simulink model "pmsg_wind_turbine"  (R2022a)
settings: Solver=ode23tb  StartTime=0.0  StopTime=30  FixedStep=1e-4  MaxStep=1e-4  RelTol=1e-3
undefined symbols (not defined in the file): Ci, kde, ke, Lb, sigbuilder_block, time, vwind
libraries: spsCurrentMeasurementLib x3, spsVoltageMeasurementLib x3, fuzblock x2, spsPWMGeneratorDCDCLib x2, eePowerMeasurement x2, spsSeriesRLCBranchLib x2, spsDCVoltageSourceLib x1, spsDiodeLib x1, spsMosfetLib x1, spsPermanentMagnetSynchronousMachineLib x1, spsThreePhaseVIMeasurementLib x1, spsUniversalBridgeLib x1
settings Model: Creator=Taysa Banik  LastModifiedBy=LICON
settings SolverCC: ZeroCrossAlgorithm=Adaptive
settings DebuggingCC: MaxConsecutiveZCsMsg=warning  MaskedZcDiagnostic=none  IgnoredZcDiagnostic=none  MultiTaskCondExecSysMsg=warning  MultiTaskRateTransMsg=warning  ModelReferenceExtraNoncontSigs=warning

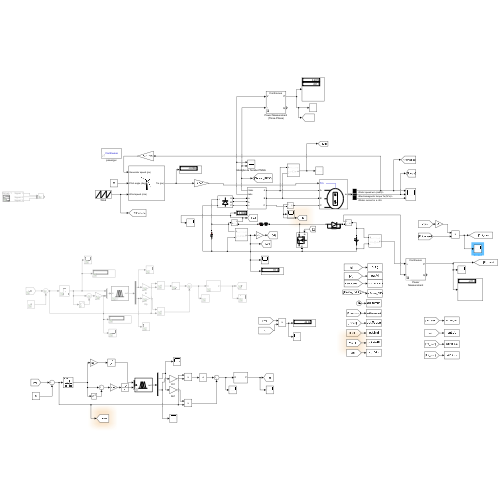
[thumbnail: Simulink's stored preview of the top-level diagram]
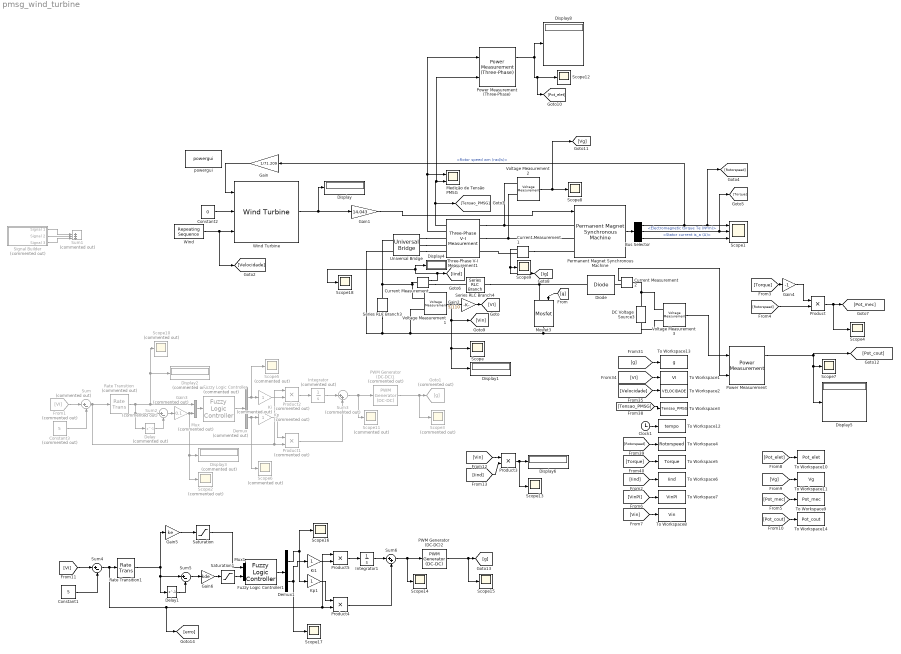
== system pmsg_wind_turbine ==
  Bus Selector : BusSelector  OutputSignals=Rotor speed wm (rad/s),Electromagnetic torque Te (N*m),Stator current is_a (A)
  Clock1 : Clock
  Constant1 : Constant  Value=5
  Constant2 : Constant  Value=0
  Constant3 : Constant  Commented=on  Value=5
  Current Measurement : spsCurrentMeasurementLib/Current Measurement  PhasorSimulation=off  OutputType=Complex  PSBequivalent=0
  Current Measurement1 : spsCurrentMeasurementLib/Current Measurement  PhasorSimulation=off  OutputType=Complex  PSBequivalent=0
  Current Measurement2 : spsCurrentMeasurementLib/Current Measurement  PhasorSimulation=off  OutputType=Complex  PSBequivalent=0
  DC Voltage Source3 : spsDCVoltageSourceLib/DC Voltage Source  Amplitude=400  Measurements=None
  Delay : Delay  Commented=on  DelayLength=1
  Delay1 : Delay  DelayLength=1
  Demux : Demux  Commented=on  Outputs=2
  Demux1 : Demux  Outputs=2
  Diode : spsDiodeLib/Diode  Ron=0.001  Lon=0  Vf=0.1  IC=0  UseSnubber=0  Rs=50000  Cs=inf  Measurements=off
  Display{,1,4..6,8} (6 alike) : Display
  Display2 : Display  Commented=on
  Display3 : Display  Commented=on
  From1 : From  Commented=on  GotoTag=VI
  Fuzzy Logic Controller : fuzblock/Fuzzy Logic  Controller  Commented=on  FIS=controladormppt  OutputSampleNumber=101  DataType=double  FuzzifiedInputs=off  RuleFiringStrengths=off  RuleOutputs=off  AggregatedOutputs=off  SimulateUsing=Interpreted execution  OutOfRangeInputValueMessage=warning  NoRuleFiredMessage=warning  EmptyOutputFuzzySetMessage=warning
  Fuzzy Logic Controller1 : fuzblock/Fuzzy Logic  Controller  FIS=controladormppt  OutputSampleNumber=101  DataType=double  FuzzifiedInputs=off  RuleFiringStrengths=off  RuleOutputs=off  AggregatedOutputs=off  SimulateUsing=Interpreted execution  OutOfRangeInputValueMessage=warning  NoRuleFiredMessage=warning  EmptyOutputFuzzySetMessage=warning
  Gain : Gain  Gain=1/71.209
  Gain1 : Gain  Gain=14.043
  Gain2 : Gain  Gain=5/110
  Gain3 : Gain  Commented=on  Gain=0.1
  Gain4 : Gain  Gain=-1
  Gain5 : Gain  Gain=ke
  Gain6 : Gain  Gain=kde
  Goto1 : Goto  Commented=on  GotoTag=g
  Integrator : Integrator  Commented=on
  Integrator1 : Integrator
  Ki : Gain  Commented=on
  Ki1 : Gain
  Kp : Gain  Commented=on
  Kp1 : Gain
  Medição de Tensão PMSG : Scope  NumInputPorts=2
  Mosfet3 : spsMosfetLib/Mosfet  Ron=0.001  Lon=0  Rd=0.01  Vfd=0  IC=0  Rs=1e5  Cs=inf  Measurements=off
  Mux : Mux  Commented=on  Inputs=2
  Mux1 : Mux  Inputs=2
  PWM Generator (DC-DC)1 : spsPWMGeneratorDCDCLib/PWM Generator (DC-DC)  Commented=on  Fsw=30000  Ts=1e-6
  PWM Generator (DC-DC)2 : spsPWMGeneratorDCDCLib/PWM Generator (DC-DC)  Fsw=30000  Ts=1e-6
  Permanent Magnet Synchronous Machine : spsPermanentMagnetSynchronousMachineLib/Permanent Magnet Synchronous Machine  NbPhases=3  FluxDistribution=Sinusoidal  RotorType=Round  MechanicalLoad=Torque Tm  PresetModel=No  ShowDetailedParameters=on  MeasurementBus=off  Resistance=0.732  Inductance=8.5e-3  dqInductances=[8.5e-3,8.5e-3]  La=3.8e-3  MachineConstant=Voltage Constant (V_peak L-L / krpm)  Flux=0.13618  VoltageCst=172.9  TorqueCst=1.4299  Flat=120  Mechanical=[1e-3 1.79E-4 7 0]  PolePairs=4  InitialConditions=[71.21,0, 0,0]  InitialConditions5ph=[0 0 0 0 0 0]  RefAngle=Aligned with phase A axis (original Park)  IterativeDiscreteModel=Trapezoidal non iterative  TsBlock=-1  TsPowergui=0
  Power Measurement : eePowerMeasurement/Power Measurement  LabelModeActiveChoice=Continuous  F=79.33  K=[0]  Ts=0
      settings: SourceProductBaseCode=PS
  Power Measurement (Three-Phase) : eePowerMeasurement/Power Measurement (Three-Phase)  LabelModeActiveChoice=Continuous  F=79.33  K=[0 1]  Seq=Positive  Ts=0
      settings: SourceProductBaseCode=PS
  Product{,3..5} (4 alike) : Product
  Product1 : Product  Commented=on
  Product2 : Product  Commented=on
  Rate Transition : RateTransition  Commented=on  OutPortSampleTime=1e-4
  Rate Transition1 : RateTransition  OutPortSampleTime=1e-4
  Saturation : Saturate  UpperLimit=1  LowerLimit=-1
  Saturation1 : Saturate  UpperLimit=1  LowerLimit=-1
  Scope{,4,7..9,12..18} (12 alike) : Scope
  Scope1 : Scope  NumInputPorts=3
  Scope{2..3,5..6,10..11} (6 alike) : Scope  Commented=on
  Series RLC Branch3 : spsSeriesRLCBranchLib/Series RLC Branch  LConnTagsString=__new0  RConnTagsString=__new0  BranchType=C  Resistance=1  Inductance=1e-3  SetiL0=off  InitialCurrent=0  Capacitance=Ci  Setx0=on  InitialVoltage=100  Measurements=None
  Series RLC Branch4 : spsSeriesRLCBranchLib/Series RLC Branch  LConnTagsString=__new0  RConnTagsString=__new0  BranchType=RL  Resistance=1  Inductance=Lb  SetiL0=off  InitialCurrent=0  Capacitance=1e-3  Setx0=off  InitialVoltage=0  Measurements=None
  Signal Builder : Subsystem  Tag=STV Subsys  Commented=on  LoadFcn=sigbuilder_block('load');  StartFcn=sigbuilder_block('start');  StopFcn=sigbuilder_block('stop');  ClipboardFcn=sigbuilder_block('clipboard');  mask(Sigbuilder block){tuvar=[0:10]}
      mask help: Simulink:masks:SigbuilderBlock_MD
      mask init:
      | if ~strcmp(get_param(bdroot(gcbh),'SimulationStatus'),'stopped') tuvar = sigbuilder_block('maskInit'); end
      settings: CopyFcn=sigbuilder_block('copy');  DeleteFcn=sigbuilder_block('delete');  ModelCloseFcn=sigbuilder_block('modelClose');  PreSaveFcn=sigbuilder_block('preSave');  PauseFcn=sigbuilder_block('pause');  ContinueFcn=sigbuilder_block('continue');  NameChangeFcn=sigbuilder_block('namechange');  OpenFcn=sigbuilder_block('open',[61.5 90 1012.5 506.25 ]);  CloseFcn=sigbuilder_block('close');
      mask Display: plot(0, 0, 100, 100,[2, 2, 32, 32, 2], [68, 8, 8, 68, 68],[32, 2], [38, 38], [32, 19, 2],[53, 60, 44], [32, 17, 17, 2],[16, 16, 31, 31]);txt = getActiveGroup(gcbh);text(2, 100, txt,'verticalAlignment', 'top');
  Sum : Sum  Commented=on  Inputs=|+-
  Sum1 : Sum  Commented=on  Inputs=|+++
  Sum2 : Sum  Commented=on  Inputs=|+-
  Sum3 : Sum  Commented=on  Inputs=|++
  Sum4 : Sum  Inputs=|+-
  Sum5 : Sum  Inputs=|+-
  Sum6 : Sum  Inputs=|++
  Three-Phase V-I Measurement1 : spsThreePhaseVIMeasurementLib/Three-Phase V-I Measurement  VoltageMeasurement=phase-to-phase  SetLabelV=off  LabelV=Vabc  Vpu=off  VpuLL=off  CurrentMeasurement=yes  SetLabelI=off  LabelI=Iabc  Ipu=off  Pbase=100e6  Vbase=500e3  OutputType=Complex  PhasorSimulation=off  PSBequivalent=0
  To Workspace1 : ToWorkspace  VariableName=VI  SampleTime=1e-6
  To Workspace10 : ToWorkspace  VariableName=Pot_elet  SampleTime=1e-6
  To Workspace11 : ToWorkspace  VariableName=Vg  SampleTime=1e-6
  To Workspace12 : ToWorkspace  VariableName=tempo  SampleTime=1e-6
  To Workspace13 : ToWorkspace  VariableName=g  SampleTime=1e-6
  To Workspace14 : ToWorkspace  VariableName=Pot_cout  SampleTime=1e-6
  To Workspace2 : ToWorkspace  VariableName=VELOCIDADE  SampleTime=1e-6
  To Workspace3 : ToWorkspace  VariableName=Tensao_PMSG  SampleTime=1e-6
  To Workspace4 : ToWorkspace  VariableName=Rotorspeed  SampleTime=1e-6
  To Workspace5 : ToWorkspace  VariableName=Torque  SampleTime=1e-6
  To Workspace6 : ToWorkspace  VariableName=Iind  SampleTime=1e-6
  To Workspace7 : ToWorkspace  VariableName=VinPI  SampleTime=1e-6
  To Workspace8 : ToWorkspace  VariableName=Vin  SampleTime=1e-6
  To Workspace9 : ToWorkspace  VariableName=Pot_mec  SampleTime=1e-6
  Universal Bridge : spsUniversalBridgeLib/Universal Bridge  Arms=3  SnubberResistance=1e5  SnubberCapacitance=inf  Device=Diodes  Ron=1e-3  Lon=0  ForwardVoltages="[  0  0  ]"  ForwardVoltage=0.1  GTOparameters=[ 10e-6 , 20e-6 ]  IGBTparameters=[ 1e-6 , 2e-6 ]  Measurements=None  Measurements_2=None  converterType=Rectifier
  Voltage Measurement1 : spsVoltageMeasurementLib/Voltage Measurement  PhasorSimulation=off  OutputType=Complex  PSBequivalent=0
  Voltage Measurement2 : spsVoltageMeasurementLib/Voltage Measurement  PhasorSimulation=off  OutputType=Complex  PSBequivalent=0
  Voltage Measurement3 : spsVoltageMeasurementLib/Voltage Measurement  PhasorSimulation=off  OutputType=Complex  PSBequivalent=0
  Wind : simulink/Sources/Repeating Sequence  rep_seq_t=[time]  rep_seq_y=[vwind]
  Wind Turbine : spsWindTurbineLib/Wind Turbine  Pnom=1000  Pelec_base=1000  wind_base=12  P_wind_base=1  speed_nom=1  pitch_angle=0  c1_c6="[0.51763          116          0.4            5           21     0.006795]"  cp_nom=0.48  lambda_nom=8.1
      settings: SourceProductBaseCode=PS
  powergui : spspowerguiLib/powergui  Priority=1  SimulationMode=Continuous  SampleTime=50e-6  frequency=60  Iterations=50  frequencyindice=0  Pbase=100e6  ErrMax=1e-4  UnitsV=kV  UnitsW=MW  buscounter=0  FunctionMessages=off  echomessages=off  EnableUseOfTLC=off  CurrentSourceSwitches=off  DisableSnubberDevices=off  DisableRonSwitches=off  DisableVfSwitches=off  DisplayEquations=off  AutomaticDiscreteSolvers=off  SolverType=Tustin/Backward Euler (TBE)  Interpol=off  ExternalGateDelay=off  methode=off  Ts=100  x0status=blocks  SPID=on  SwTol=0  HookPort=off  NonlinearTolerance=1e-4  nMaxIteration=100  ContinueOnMaxIteration=off  RestoreLinks=warning  ResistiveCurrentMeasurement=off  Frange=[0:2:500]  Ylog=off  Xlog=on  ShowGrid=off  save=off  variable=ZData  structure=0  ZoomFFT=off  StartTime=0.0  cycles=1  DisplayStyle=1  fundamental=60  FreqAxis=off  MaxFrequency=1000  frequencyindicesteady=1  RmsSteady=1  display=off
  wires:
  Constant2/1 -> Wind Turbine/2
  Three-Phase V-I Measurement1/1 -> Power Measurement (Three-Phase)/2, Medição de Tensão PMSG/2, [Tensao_PMSG]
  Three-Phase V-I Measurement1/2 -> Power Measurement (Three-Phase)/1, Medição de Tensão PMSG/1
  Permanent Magnet Synchronous Machine/1 -> Bus Selector/1
  Bus Selector/1 -> Scope1/1, [Rotorspeed], Gain/1  "<Rotor speed wm (rad/s)>"
  Bus Selector/2 -> [Torque], Scope1/2  "<Electromagnetic torque Te (N*m)>"
  Bus Selector/3 -> Scope1/3  "<Stator current is_a (A)>"
  Gain/1 -> Wind Turbine/1
  Wind Turbine/1 -> Display/1, Gain1/1
  Gain1/1 -> Permanent Magnet Synchronous Machine/1
  Voltage Measurement1/1 -> Gain2/1, Scope/1, Display1/1, [Vin]
  [g] -> Mosfet3/1
  From1/1 -> Sum/1
  Constant3/1 -> Sum/2
  PWM Generator (DC-DC)1/1 -> Scope3/1, Goto1/1
  Gain2/1 -> [VI]
  Signal Builder/1(Signal 1) -> Sum1/1
  Signal Builder/2(Signal 2) -> Sum1/2
  Signal Builder/3(Signal 3) -> Sum1/3
  [VI] -> To Workspace1/1
  [g] -> To Workspace13/1
  [Torque] -> To Workspace5/1
  [Velocidade] -> To Workspace2/1
  Clock1/1 -> To Workspace12/1
  [Tensao_PMSG] -> To Workspace3/1
  [Rotorspeed] -> To Workspace4/1
  Current Measurement/1 -> Scope18/1, Display4/1, [Iind]
  [Iind] -> To Workspace6/1
  Product/1 -> Scope4/1, [Pot_mec]
  [Rotorspeed] -> Product/2
  [Torque] -> Gain4/1
  Gain4/1 -> Product/1
  Sum/1 -> Rate Transition/1, Product2/1, Product1/2
  Demux/2 -> Scope6/1, Kp/1
  Kp/1 -> Product1/1
  Demux/1 -> Scope5/1, Ki/1
  Ki/1 -> Product2/2
  Product2/1 -> Integrator/1
  Integrator/1 -> Sum3/1
  Product1/1 -> Sum3/2
  Sum3/1 -> Scope11/1, PWM Generator (DC-DC)1/1
  Mux/1 -> Fuzzy Logic Controller/1
  Fuzzy Logic Controller/1 -> Demux/1
  [VinPI] -> To Workspace7/1
  [Vin] -> To Workspace8/1
  [Pot_mec] -> To Workspace9/1
  [Pot_elet] -> To Workspace10/1
  Voltage Measurement2/1 -> [Vg], Scope8/1
  Current Measurement1/1 -> [Ig], Scope9/1
  [Vg] -> To Workspace11/1
  Power Measurement (Three-Phase)/1 -> [Pot_elet], Scope12/1, Display8/1
  Power Measurement/1 -> Display5/1, Scope7/1, [Pot_cout]
  Voltage Measurement3/1 -> Power Measurement/1
  Current Measurement2/1 -> Power Measurement/2
  [Pot_cout] -> To Workspace14/1
  Gain3/1 -> Scope2/1, Display3/1, Mux/2
  Rate Transition/1 -> Delay/1, Sum2/1, Scope10/1, Display2/1, Mux/1
  Sum2/1 -> Gain3/1
  Delay/1 -> Sum2/2
  [Iind] -> Product3/2
  Product3/1 -> Scope13/1, Display6/1
  [Vin] -> Product3/1
  Saturation1/1 -> Mux1/2
  Sum5/1 -> Gain6/1
  Delay1/1 -> Sum5/2
  Integrator1/1 -> Sum6/1
  Mux1/1 -> Fuzzy Logic Controller1/1
  Demux1/1 -> Kp1/1, Scope16/1
  Gain5/1 -> Saturation/1
  Ki1/1 -> Product5/2
  Sum6/1 -> Scope14/1, PWM Generator (DC-DC)2/1
  Rate Transition1/1 -> Gain5/1, Delay1/1, Sum5/1
  Constant1/1 -> Sum4/2
  [VI] -> Sum4/1
  Demux1/2 -> Ki1/1, Scope17/1
  PWM Generator (DC-DC)2/1 -> Scope15/1, [g]
  Product5/1 -> Integrator1/1
  Sum4/1 -> Rate Transition1/1, [erro], Product5/1, Product4/2
  Saturation/1 -> Mux1/1
  Gain6/1 -> Saturation1/1
  Kp1/1 -> Product4/1
  Product4/1 -> Sum6/2
  Fuzzy Logic Controller1/1 -> Demux1/1
  Wind/1 -> [Velocidade], Wind Turbine/3
  connections:
  Three-Phase V-I Measurement1/LConn1 -- Voltage Measurement2/LConn1 -- Permanent Magnet Synchronous Machine/LConn1
  Three-Phase V-I Measurement1/LConn2 -- Voltage Measurement2/LConn2 -- Permanent Magnet Synchronous Machine/LConn2
  Universal Bridge/LConn1 -- Three-Phase V-I Measurement1/RConn1
  Universal Bridge/LConn2 -- Three-Phase V-I Measurement1/RConn2
  Universal Bridge/LConn3 -- Three-Phase V-I Measurement1/RConn3
  Mosfet3/LConn1 -- Diode/LConn1 -- Series RLC Branch4/RConn1
  Voltage Measurement1/LConn1 -- Current Measurement/LConn1 -- Universal Bridge/RConn1 -- Series RLC Branch3/LConn1
  Series RLC Branch3/RConn1 -- Universal Bridge/RConn2 -- Voltage Measurement1/LConn2 -- Voltage Measurement3/LConn2 -- DC Voltage Source3/LConn1 -- Mosfet3/RConn1
  DC Voltage Source3/RConn1 -- Current Measurement2/LConn1 -- Voltage Measurement3/LConn1
  Current Measurement1/LConn1 -- Permanent Magnet Synchronous Machine/LConn3
  Current Measurement1/RConn1 -- Three-Phase V-I Measurement1/LConn3
  Current Measurement2/RConn1 -- Diode/RConn1
  Current Measurement/RConn1 -- Series RLC Branch4/LConn1

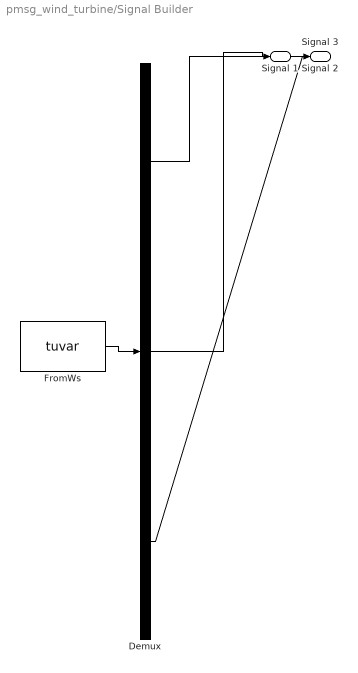
== system pmsg_wind_turbine/Signal Builder ==
  Demux : Demux  Tag=STV Demux  Outputs=3
      settings: DisplayOption=none
  FromWs : FromWorkspace  Tag=STV FromWs  VariableName=tuvar
      SigBuilderData=|
      | common.afterFinalStr = 'Extrapolate'
      | common.sampleTime = 0
      | dataSet.timeRange = [0 10]
      | dataSet.name = 'Group 1'
      | sbobj.Groups.Name = 'Group 1'
      | sbobj.Groups.Signals(1).Name = 'Signal 1'
      | sbobj.Groups.Signals(1).XData = [0 1.5 1.5 6 10]
      | sbobj.Groups.Signals(1).YData = [12 12 0 0 0]
      | sbobj.Groups.Signals(2).Name = 'Signal 2'
      | sbobj.Groups.Signals(2).XData = [0 1.5 1.5 2.5 2.5 10]
      | sbobj.Groups.Signals(2).YData = [0 0 10 10 0 0]
      | sbobj.Groups.Signals(3).Name = 'Signal 3'
      | sbobj.Groups.Signals(3).XData = [0 2.5 2.5 10]
      | sbobj.Groups.Signals(3).YData = [0 0 12 12]
  Signal 1 : Outport  Tag=STV Outport
  Signal 2 : Outport  Tag=STV Outport  Port=2
  Signal 3 : Outport  Tag=STV Outport  Port=3
  wires:
  Demux/1 -> Signal 1/1
  FromWs/1 -> Demux/1
  Demux/2 -> Signal 2/1
  Demux/3 -> Signal 3/1
